simulink library "PM100DX"  (R2025a)
settings: Solver=VariableStepAuto  StartTime=0.0  StopTime=10.0  RelTol=1e-3
undefined symbols (not defined in the file or in its folder): raptor_xcp_function, StateCAN
libraries: Utilities x15, Raptor_lib x7, simulink x1
settings Model: Creator=serga  LastModifiedBy=hyuga

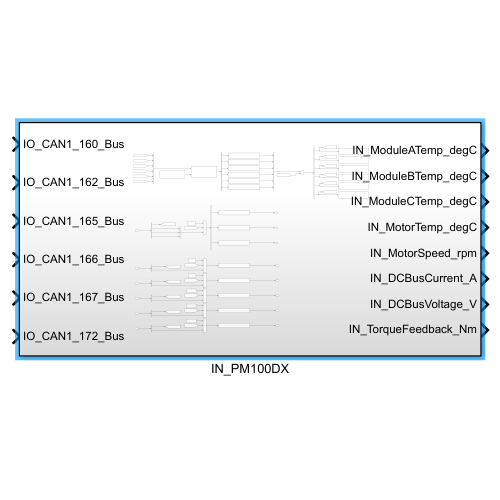
[thumbnail: Simulink's stored preview of the top-level diagram]
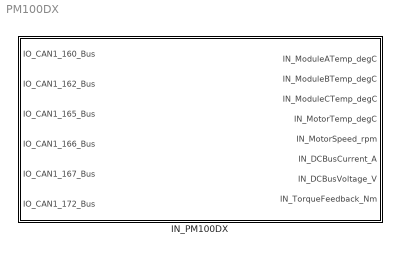
== system PM100DX ==
  IN_PM100DX : Subsystem

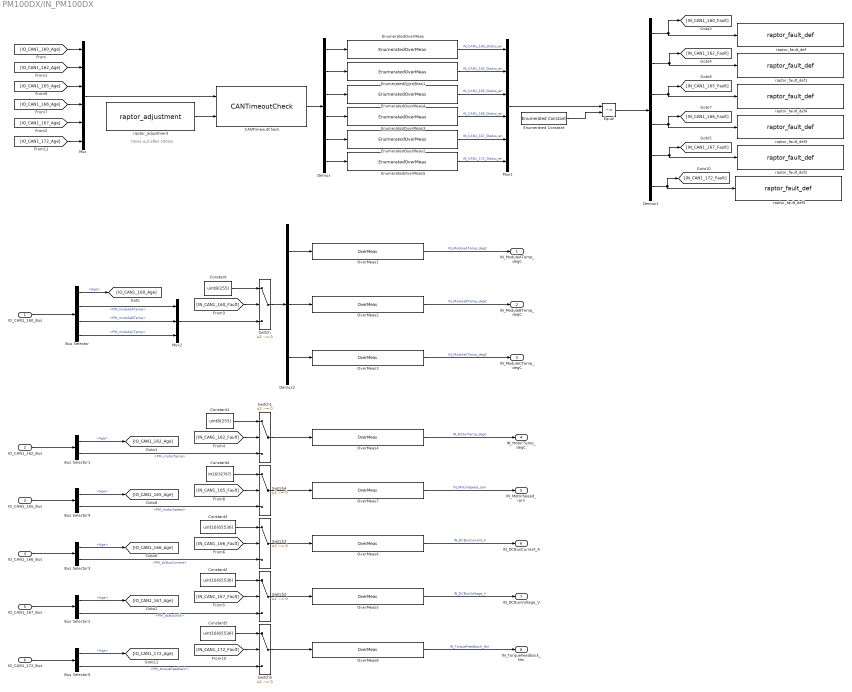
== system PM100DX/IN_PM100DX ==
  note: times out after 100ms
  IO_CAN1_160_Bus : Inport
  IO_CAN1_162_Bus : Inport  Port=2
  IO_CAN1_165_Bus : Inport  Port=3
  IO_CAN1_166_Bus : Inport  Port=4
  IO_CAN1_167_Bus : Inport  Port=5
  IO_CAN1_172_Bus : Inport  Port=6
  Bus Selector : BusSelector  OutputSignals=Age,PM_moduleATemp,PM_moduleBTemp,PM_moduleCTemp
  Bus Selector1 : BusSelector  OutputSignals=Age,PM_motorTemp
  Bus Selector2 : BusSelector  OutputSignals=Age,PM_dcBusVolt
  Bus Selector3 : BusSelector  OutputSignals=Age,PM_dcBusCurrent
  Bus Selector4 : BusSelector  OutputSignals=Age,PM_motorSpeed
  Bus Selector5 : BusSelector  OutputSignals=Age,PM_torqueFeedback
  CANTimeoutCheck : Utilities/CANTimeoutCheck
  Constant : Constant  Value=uint8(255)
  Constant1 : Constant  Value=uint8(255)
  Constant2 : Constant  Value=uint16(65536)
  Constant3 : Constant  Value=uint16(65536)
  Constant4 : Constant  Value=int16(32767)
  Constant5 : Constant  Value=uint16(65536)
  Demux : Demux  Outputs=6
  Demux1 : Demux  Outputs=6
  Demux2 : Demux  Outputs=3
  Enumerated Constant : simulink/Sources/Enumerated Constant  OutDataTypeStr=Enum: StateCAN  Value=StateCAN.Normal  SampleTime=inf
  EnumeratedOverMeas : Utilities/EnumeratedOverMeas  sigName='IN_CAN1_160_Status_en'  enumName='StateCAN'
  EnumeratedOverMeas1 : Utilities/EnumeratedOverMeas  sigName='IN_CAN1_162_Status_en'  enumName='StateCAN'
  EnumeratedOverMeas2 : Utilities/EnumeratedOverMeas  sigName='IN_CAN1_167_Status_en'  enumName='StateCAN'
  EnumeratedOverMeas3 : Utilities/EnumeratedOverMeas  sigName='IN_CAN1_166_Status_en'  enumName='StateCAN'
  EnumeratedOverMeas4 : Utilities/EnumeratedOverMeas  sigName='IN_CAN1_165_Status_en'  enumName='StateCAN'
  EnumeratedOverMeas5 : Utilities/EnumeratedOverMeas  sigName='IN_CAN1_172_Status_en'  enumName='StateCAN'
  Equal : RelationalOperator  Operator=~=  OutDataTypeStr=boolean  RndMeth=Simplest  InputSameDT=off
  Mux : Mux  Inputs=6
  Mux1 : Mux  Inputs=6
  Mux2 : Mux  Inputs=3
  OverMeas1 : Utilities/OverMeas  sigName='IN_ModuleATemp_degC'  minimum=-inf  maximum=inf
  OverMeas2 : Utilities/OverMeas  sigName='IN_ModuleBTemp_degC'  minimum=-inf  maximum=inf
  OverMeas3 : Utilities/OverMeas  sigName='IN_ModuleCTemp_degC'  minimum=-inf  maximum=inf
  OverMeas4 : Utilities/OverMeas  sigName='IN_MotorTemp_degC'  minimum=-inf  maximum=inf
  OverMeas5 : Utilities/OverMeas  sigName='IN_DCBusVoltage_V'  minimum=-inf  maximum=inf
  OverMeas6 : Utilities/OverMeas  sigName='IN_DCBusCurrent_A'  minimum=-inf  maximum=inf
  OverMeas7 : Utilities/OverMeas  sigName='IN_MotorSpeed_rpm'  minimum=-inf  maximum=inf
  OverMeas8 : Utilities/OverMeas  sigName='IN_TorqueFeedback_Nm'  minimum=-inf  maximum=inf
  Switch{,1..5} (6 alike) : Switch  Criteria=u2 ~= 0  SaturateOnIntegerOverflow=off  InputSameDT=off
  raptor_adjustment : Raptor_lib/Data Storage/raptor_adjustment  paramName='IN_PM100DXTOThresh_na'  nameSource=Parameter  initValue=20  dataType=uint32  storage=Calibration  calDispType=Number  calEnum={'False', 'True'}  calGain=1.0  calOffset=0.0  calMax=inf  calMin=-inf  calFormat='-1'  calUnit=''  calHelp=''  calAccess=1  calFunction=raptor_xcp_function(gcb)  calDispHeaders=off  calColHeaders={'Col1' 'Col2' 'Col3'}  calRowHeaders={'Row1' 'Row2' 'Row3'}
      settings: SourceProductName=Raptor
  raptor_fault_def : Raptor_lib/Faults/raptor_fault_def  faultName='IN_CAN1_160_Fault'  persist=on  sticky=off  emisRelated=off  permanent=off  singleTrip=off  clearMethod=Standard  xLimit=25  yLimit=50  calEnable=on  addDisable=off  calAccess=1  calFunction='System | FaultManager'
      settings: SourceProductName=Raptor
  raptor_fault_def1 : Raptor_lib/Faults/raptor_fault_def  faultName='IN_CAN1_162_Fault'  persist=on  sticky=off  emisRelated=off  permanent=off  singleTrip=off  clearMethod=Standard  xLimit=25  yLimit=50  calEnable=on  addDisable=off  calAccess=1  calFunction='System | FaultManager'
      settings: SourceProductName=Raptor
  raptor_fault_def2 : Raptor_lib/Faults/raptor_fault_def  faultName='IN_CAN1_167_Fault'  persist=on  sticky=off  emisRelated=off  permanent=off  singleTrip=off  clearMethod=Standard  xLimit=25  yLimit=50  calEnable=on  addDisable=off  calAccess=1  calFunction='System | FaultManager'
      settings: SourceProductName=Raptor
  raptor_fault_def3 : Raptor_lib/Faults/raptor_fault_def  faultName='IN_CAN1_166_Fault'  persist=on  sticky=off  emisRelated=off  permanent=off  singleTrip=off  clearMethod=Standard  xLimit=25  yLimit=50  calEnable=on  addDisable=off  calAccess=1  calFunction='System | FaultManager'
      settings: SourceProductName=Raptor
  raptor_fault_def4 : Raptor_lib/Faults/raptor_fault_def  faultName='IN_CAN1_165_Fault'  persist=on  sticky=off  emisRelated=off  permanent=off  singleTrip=off  clearMethod=Standard  xLimit=25  yLimit=50  calEnable=on  addDisable=off  calAccess=1  calFunction='System | FaultManager'
      settings: SourceProductName=Raptor
  raptor_fault_def5 : Raptor_lib/Faults/raptor_fault_def  faultName='IN_CAN1_172_Fault'  persist=on  sticky=off  emisRelated=off  permanent=off  singleTrip=off  clearMethod=Standard  xLimit=25  yLimit=50  calEnable=on  addDisable=off  calAccess=1  calFunction='System | FaultManager'
      settings: SourceProductName=Raptor
  IN_ModuleATemp_degC : Outport
  IN_ModuleBTemp_degC : Outport  Port=2
  IN_ModuleCTemp_degC : Outport  Port=3
  IN_MotorTemp_degC : Outport  Port=4
  IN_MotorSpeed_rpm : Outport  Port=5
  IN_DCBusCurrent_A : Outport  Port=6
  IN_DCBusVoltage_V : Outport  Port=7
  IN_TorqueFeedback_Nm : Outport  Port=8
  wires:
  Demux2/1 -> OverMeas1/1
  Demux2/3 -> OverMeas3/1
  Demux2/2 -> OverMeas2/1
  Bus Selector/4 -> Mux2/3  "<PM_moduleCTemp>"
  Bus Selector/3 -> Mux2/2  "<PM_moduleBTemp>"
  Bus Selector/2 -> Mux2/1  "<PM_moduleATemp>"
  OverMeas1/1 -> IN_ModuleATemp_degC/1  "IN_ModuleATemp_degC"
  OverMeas3/1 -> IN_ModuleCTemp_degC/1  "IN_ModuleCTemp_degC"
  OverMeas2/1 -> IN_ModuleBTemp_degC/1  "IN_ModuleBTemp_degC"
  Demux1/4 -> [IN_CAN1_166_Fault], raptor_fault_def3/1
  EnumeratedOverMeas3/1 -> Mux1/4  "IN_CAN1_166_Status_en"
  Demux/4 -> EnumeratedOverMeas3/1
  [IO_CAN1_166_Age] -> Mux/4
  OverMeas6/1 -> IN_DCBusCurrent_A/1  "IN_DCBusCurrent_A"
  Switch3/1 -> OverMeas6/1
  Constant3/1 -> Switch3/1
  [IN_CAN1_166_Fault] -> Switch3/2
  Bus Selector3/1 -> [IO_CAN1_166_Age]  "<Age>"
  IO_CAN1_166_Bus/1 -> Bus Selector3/1
  Switch2/1 -> OverMeas5/1
  IO_CAN1_167_Bus/1 -> Bus Selector2/1
  IO_CAN1_162_Bus/1 -> Bus Selector1/1
  IO_CAN1_160_Bus/1 -> Bus Selector/1
  Bus Selector/1 -> [IO_CAN1_160_Age]  "<Age>"
  Bus Selector1/1 -> [IO_CAN1_162_Age]  "<Age>"
  Bus Selector1/2 -> Switch1/3  "<PM_motorTemp>"
  Bus Selector2/1 -> [IO_CAN1_167_Age]  "<Age>"
  Bus Selector2/2 -> Switch2/3  "<PM_dcBusVolt>"
  Mux/1 -> CANTimeoutCheck/1
  [IO_CAN1_160_Age] -> Mux/1
  [IO_CAN1_162_Age] -> Mux/2
  [IO_CAN1_167_Age] -> Mux/5
  raptor_adjustment/1 -> CANTimeoutCheck/2
  CANTimeoutCheck/1 -> Demux/1
  Enumerated Constant/1 -> Equal/2
  Demux/1 -> EnumeratedOverMeas/1
  Demux/2 -> EnumeratedOverMeas1/1
  Demux/3 -> EnumeratedOverMeas4/1
  EnumeratedOverMeas/1 -> Mux1/1  "IN_CAN1_160_Status_en"
  EnumeratedOverMeas1/1 -> Mux1/2  "IN_CAN1_162_Status_en"
  EnumeratedOverMeas2/1 -> Mux1/5  "IN_CAN1_167_Status_en"
  Mux1/1 -> Equal/1
  Equal/1 -> Demux1/1
  Demux1/1 -> raptor_fault_def/1, [IN_CAN1_160_Fault]
  Demux1/2 -> [IN_CAN1_162_Fault], raptor_fault_def1/1
  Demux1/5 -> [IN_CAN1_167_Fault], raptor_fault_def2/1
  Mux2/1 -> Switch/3
  [IN_CAN1_160_Fault] -> Switch/2
  Constant/1 -> Switch/1
  Switch/1 -> Demux2/1
  [IN_CAN1_162_Fault] -> Switch1/2
  Constant1/1 -> Switch1/1
  Switch1/1 -> OverMeas4/1
  OverMeas4/1 -> IN_MotorTemp_degC/1  "IN_MotorTemp_degC"
  [IN_CAN1_167_Fault] -> Switch2/2
  Constant2/1 -> Switch2/1
  OverMeas5/1 -> IN_DCBusVoltage_V/1  "IN_DCBusVoltage_V"
  Bus Selector3/2 -> Switch3/3  "<PM_dcBusCurrent>"
  IO_CAN1_165_Bus/1 -> Bus Selector4/1
  Bus Selector4/1 -> [IO_CAN1_165_Age]  "<Age>"
  Bus Selector4/2 -> Switch4/3  "<PM_motorSpeed>"
  Switch4/1 -> OverMeas7/1
  [IN_CAN1_165_Fault] -> Switch4/2
  Constant4/1 -> Switch4/1
  OverMeas7/1 -> IN_MotorSpeed_rpm/1  "IN_MotorSpeed_rpm"
  [IO_CAN1_165_Age] -> Mux/3
  Demux/5 -> EnumeratedOverMeas2/1
  EnumeratedOverMeas4/1 -> Mux1/3  "IN_CAN1_165_Status_en"
  Demux1/3 -> [IN_CAN1_165_Fault], raptor_fault_def4/1
  OverMeas8/1 -> IN_TorqueFeedback_Nm/1  "IN_TorqueFeedback_Nm"
  Constant5/1 -> Switch5/1
  [IN_CAN1_172_Fault] -> Switch5/2
  Switch5/1 -> OverMeas8/1
  Bus Selector5/2 -> Switch5/3  "<PM_torqueFeedback>"
  IO_CAN1_172_Bus/1 -> Bus Selector5/1
  Bus Selector5/1 -> [IO_CAN1_172_Age]  "<Age>"
  [IO_CAN1_172_Age] -> Mux/6
  Demux/6 -> EnumeratedOverMeas5/1
  EnumeratedOverMeas5/1 -> Mux1/6  "IN_CAN1_172_Status_en"
  Demux1/6 -> raptor_fault_def5/1, [IN_CAN1_172_Fault]
